simulink model "ControleOtimo_simulink"  (R2019a)
settings: Solver=FixedStepAuto  StartTime=0.0  StopTime=10  FixedStep=0.05  RelTol=1e-3  EnableMultiTasking=on
values from neighbouring files (symbols this model uses):
  K = lqr(A,B,Q,R)    [ControleOtimo.m]    (also in Identif_CecilSmith.m = yfinal/Degrau(end); Identif_Sundaresan.m = yfinal/Degrau(end); Retroacao_de_estados_1a_Lei.m = acker(a,b,J); Retroacao_de_estados_2a_Lei.m = acker(a,b,J))
settings Model: Creator=Joao Paulo  LastModifiedBy=vinic
settings DataIOCC: LimitDataPoints=on  SaveFormat=Array  ReturnWorkspaceOutputs=off
settings OptimizationCC: ExpressionDepthLimit=2147483647  LifeSpan=inf
settings DebuggingCC: UnderspecifiedInitializationDetection=Classic  MergeDetectMultiDrivingBlocksExec=none  SolverPrmCheckMsg=warning  StateNameClashWarn=warning  SFUnexpectedBacktrackingDiag=warning  SFNoUnconditionalDefaultTransitionDiag=warning  SFExecutionAtInitializationDiag=none  ArithmeticOperatorsInVariantConditions=warning
settings HardwareCC: ProdBitPerPointer=32  ProdBitPerSizeT=32  ProdBitPerPtrDiffT=32  ProdLargestAtomicFloat=None  ProdIntDivRoundTo=Undefined  ProdEndianess=Unspecified  ProdWordSize=32  ProdHWDeviceType=32-bit Generic
settings ModelReferenceCC: PropagateSignalLabelsOutOfModel=off
settings SFSimCC: SimUseLocalCustomCode=off
settings RTWCC: RTWUseLocalCustomCode=off
settings CodeAppCC: StateflowObjectComments=on
settings GRTTargetCC: TargetLangStandard=C89/C90 (ANSI)  GeneratePreprocessorConditionals=Disable all
settings ConfigComp: CovMetricSettings=dw  CovHtmlReporting=on  CovSaveCumulativeToWorkspaceVar=on  CovSaveSingleToWorkspaceVar=on  CovExternalEMLEnable=off

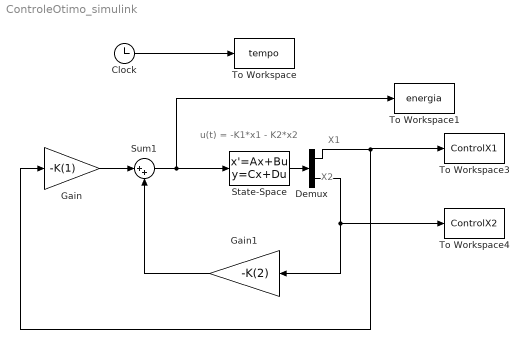
== system ControleOtimo_simulink ==
  note: u(t) = -K1*x1 - K2*x2
  note: X2
  note: X1
  Clock : Clock
  Demux : Demux  Outputs=2
  Gain : Gain  Gain=-K(1)
  Gain1 : Gain  Gain=-K(2)
  State-Space : StateSpace  A=[0 1; 0.01 0]  B=[0; 1]  C=[1 0; 0 1]  D=[0 ;0]  InitialCondition=[3;0]
  Sum1 : Sum  Inputs=|++
  To Workspace : ToWorkspace  VariableName=tempo  SampleTime=-1
  To Workspace1 : ToWorkspace  VariableName=energia  SampleTime=-1
  To Workspace3 : ToWorkspace  VariableName=ControlX1  SampleTime=-1
  To Workspace4 : ToWorkspace  VariableName=ControlX2  SampleTime=-1
  wires:
  Clock/1 -> To Workspace/1
  Gain/1 -> Sum1/1
  Sum1/1 -> To Workspace1/1, State-Space/1
  Gain1/1 -> Sum1/2
  State-Space/1 -> Demux/1
  Demux/1 -> To Workspace3/1, Gain/1
  Demux/2 -> To Workspace4/1, Gain1/1
